simulink model "skysurfer_controller_with_integral_action"  (R2021a)
settings: Solver=VariableStepAuto  StartTime=0.0  StopTime=100  RelTol=1e-3
values from neighbouring files (symbols this model uses):
  D = [0;0;0;0]    [skysurfer_controller.m]
undefined symbols (not defined in the file or in its folder): Aaug, Baug, Caug, k1
libraries: cstblocks x1
settings Model: Creator=astik  LastModifiedBy=astik

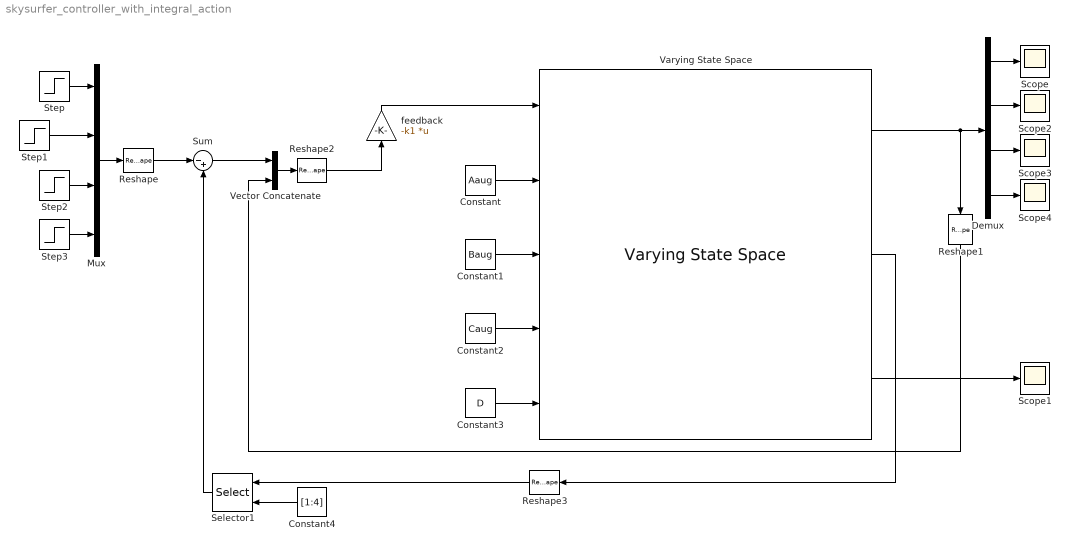
== system skysurfer_controller_with_integral_action ==
  Constant : Constant  Value=Aaug
  Constant1 : Constant  Value=Baug
  Constant2 : Constant  Value=Caug
  Constant3 : Constant  Value=D
  Constant4 : Constant  Value=[1:4]
  Demux : Demux
  Mux : Mux
  Reshape{,1..3} (4 alike) : Reshape  OutputDimensionality=Column vector (2-D)
  Scope{,1..4} (5 alike) : Scope
  Selector1 : Selector  InputPortWidth=8  IndexOptions=Index vector (port)  Indices=[1 5]  OutputSizes=1
  Step : Step  Time=4  After=30  SampleTime=0
  Step1 : Step  Time=2  After=0  SampleTime=0
  Step2 : Step  After=0  SampleTime=0
  Step3 : Step  After=0.51  SampleTime=0
  Sum : Sum  Inputs=|-+
  Varying State Space : cstblocks/Linear Parameter Varying/Varying State Space  x0=1  xNames=''  OutputX=on  OutputDX=on
  Vector Concatenate : Concatenate
  feedback : Gain  Gain=-k1  Multiplication=Matrix(K*u)
  wires:
  Mux/1 -> Reshape/1
  Step/1 -> Mux/1
  Varying State Space/1 -> Demux/1, Reshape1/1
  Demux/4 -> Scope4/1
  Demux/3 -> Scope3/1
  Demux/1 -> Scope/1
  feedback/1 -> Varying State Space/1
  Demux/2 -> Scope2/1
  Varying State Space/2 -> Reshape3/1
  Constant/1 -> Varying State Space/2
  Step1/1 -> Mux/2
  Constant2/1 -> Varying State Space/4
  Constant1/1 -> Varying State Space/3
  Constant3/1 -> Varying State Space/5
  Step3/1 -> Mux/4
  Step2/1 -> Mux/3
  Reshape/1 -> Sum/1
  Varying State Space/3 -> Scope1/1
  Sum/1 -> Vector Concatenate/1
  Reshape1/1 -> Vector Concatenate/2
  Vector Concatenate/1 -> Reshape2/1
  Reshape2/1 -> feedback/1
  Selector1/1 -> Sum/2
  Constant4/1 -> Selector1/2
  Reshape3/1 -> Selector1/1
